simulink model "MPPT"  (R2024b)
settings: Solver=FixedStepAuto  StartTime=0.0  StopTime=1  FixedStep=Ts  RelTol=1e-3
InitFcn:
  | Ts = 1e-6;
  | N = 1000;
  | A = -0.001;
  | B = 0.001
libraries: simulink x9, spsSeriesRLCBranchLib x4, spsCurrentMeasurementLib x1, spsDiodeLib x1, spsMosfetLib x1, spsPVArrayLib x1, spsVoltageMeasurementLib x1, sps_lib x1
settings Model: Creator=Ketan  LastModifiedBy=Ketan

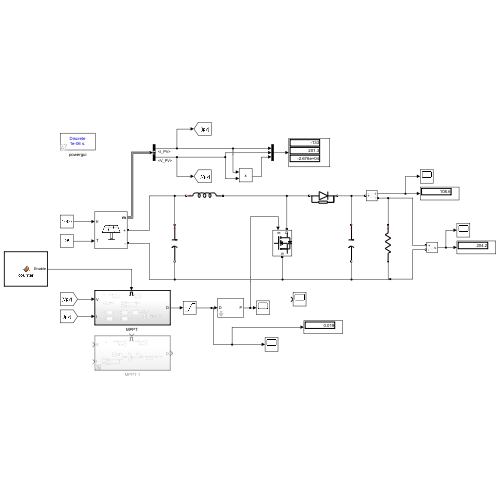
[thumbnail: Simulink's stored preview of the top-level diagram]
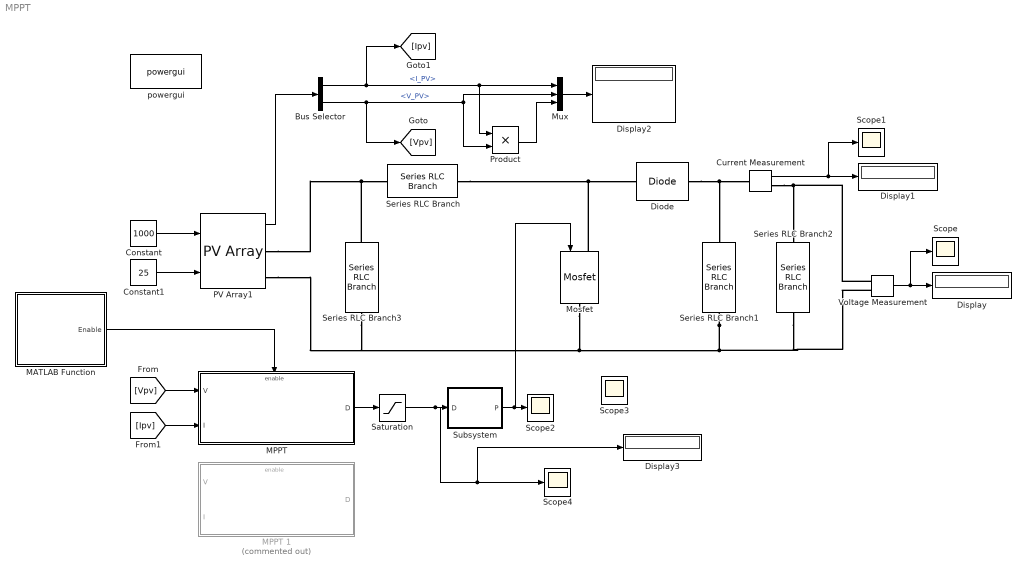
== system MPPT ==
  Bus Selector : BusSelector  OutputSignals=I_PV,V_PV
  Constant : Constant  Value=1000
  Constant1 : Constant  Value=25
  Current Measurement : spsCurrentMeasurementLib/Current Measurement  PhasorSimulation=off  OutputType=Complex  PSBequivalent=0
  Diode : spsDiodeLib/Diode  Ron=0.001  Lon=0  Vf=0.8  IC=0  UseSnubber=0  Rs=500  Cs=250e-9  Measurements=off
  Display{,1..3} (4 alike) : Display
  MATLAB Function : MATLAB Function  TreatAsAtomicUnit=on
  "MPPT " : Subsystem
  MPPT 1 : Subsystem  Commented=on
  Mosfet : spsMosfetLib/Mosfet  Ron=0.1  Lon=0  Rd=0.01  Vfd=0  IC=0  Rs=1e5  Cs=inf  Measurements=off
  Mux : Mux  Inputs=3
  PV Array1 : spsPVArrayLib/PV Array  Npar=40  Nser=10  PlotType=array @ 1000 W/m2 & specified temperatures  S_vec="[ 1000  500  100 ]"  Temp_C_vec="[ 45 25  ]"  ModuleName=User-defined  PlotWhenSelected=off  Pm=213.15  Ncell=60  Voc=36.3  Isc=7.84  Vm=29  Im=7.35  beta_Voc_pc=-0.36099  alpha_Isc_pc=0.102  beta_Voc=-0.13104  alpha_Isc=0.0079968  IL=7.8654  I0=2.9273e-10  nI=0.98119  Rsh=313.0553  Rs=0.39381  RobustModel=off  RobustCellTemperature=313.3991  BAL=on  Tc=1e-6  Tfilter=5e-5
  Product : Product
  Saturation : Saturate  UpperLimit=0.9  LowerLimit=0.005
  Scope{,1..4} (5 alike) : Scope
  Series RLC Branch : spsSeriesRLCBranchLib/Series RLC Branch  LConnTagsString=__new0  RConnTagsString=__new0  BranchType=L  Resistance=1  Inductance=45e-6  SetiL0=off  InitialCurrent=0  Capacitance=1e-6  Setx0=off  InitialVoltage=0  Measurements=None
  Series RLC Branch1 : spsSeriesRLCBranchLib/Series RLC Branch  LConnTagsString=__new0  RConnTagsString=__new0  BranchType=C  Resistance=1  Inductance=1e-3  SetiL0=off  InitialCurrent=0  Capacitance=244e-6  Setx0=off  InitialVoltage=400  Measurements=None
  Series RLC Branch2 : spsSeriesRLCBranchLib/Series RLC Branch  LConnTagsString=__new0  RConnTagsString=__new0  BranchType=R  Resistance=1.88  Inductance=1e-3  SetiL0=off  InitialCurrent=0  Capacitance=1e-6  Setx0=off  InitialVoltage=0  Measurements=None
  Series RLC Branch3 : spsSeriesRLCBranchLib/Series RLC Branch  LConnTagsString=__new0  RConnTagsString=__new0  BranchType=C  Resistance=1  Inductance=1e-3  SetiL0=off  InitialCurrent=0  Capacitance=100e-6  Setx0=off  InitialVoltage=0  Measurements=None
  Subsystem : Subsystem  mask{fs=20000}
      mask prompts: fs "Frequency"
      mask DialogControl DescTextVar Prompt: This Block Genertates a PWM signal based on the Frequency of Carrier Wave and Duty Cycle
  Voltage Measurement : spsVoltageMeasurementLib/Voltage Measurement  PhasorSimulation=off  OutputType=Complex  PSBequivalent=0
  powergui : sps_lib/powergui  Priority=1  SimulationMode=Discrete  SampleTime=Ts  frequency=60  Iterations=50  frequencyindice=0  Pbase=100e6  ErrMax=1e-4  UnitsV=kV  UnitsW=MW  buscounter=0  FunctionMessages=off  echomessages=off  EnableUseOfTLC=off  CurrentSourceSwitches=off  DisableSnubberDevices=off  DisableRonSwitches=off  DisableVfSwitches=off  DisplayEquations=off  AutomaticDiscreteSolvers=off  SolverType=Tustin/Backward Euler (TBE)  Interpol=off  ExternalGateDelay=off  methode=off  Ts=100  x0status=blocks  SPID=on  SwTol=0  HookPort=off  NonlinearTolerance=1e-4  nMaxIteration=100  ContinueOnMaxIteration=off  RestoreLinks=warning  ResistiveCurrentMeasurement=off  Frange=[0:2:500]  Ylog=off  Xlog=on  ShowGrid=off  save=off  variable=ZData  structure=0  ZoomFFT=off  StartTime=0.0  cycles=1  DisplayStyle=1  fundamental=60  FreqAxis=off  MaxFrequency=1000  frequencyindicesteady=1  RmsSteady=1  display=off
  wires:
  Voltage Measurement/1 -> Scope/1, Display/1
  Subsystem/1(P) -> Mosfet/1, Scope2/1
  Constant/1 -> PV Array1/1
  Constant1/1 -> PV Array1/2
  PV Array1/1 -> Bus Selector/1
  Mux/1 -> Display2/1
  Current Measurement/1 -> Scope1/1, Display1/1
  Saturation/1 -> Display3/1, Scope4/1, Subsystem/1(D)
  Bus Selector/1 -> [Ipv], Product/1, Mux/1  "<I_PV>"
  Bus Selector/2 -> [Vpv], Product/2, Mux/2  "<V_PV>"
  "MPPT "/1(D) -> Saturation/1
  MATLAB Function/1(Enable) -> "MPPT "/Enable
  [Vpv] -> "MPPT "/1(V)
  [Ipv] -> "MPPT "/2(I)
  Product/1 -> Mux/3
  connections:
  Series RLC Branch1/RConn1 -- Voltage Measurement/LConn2 -- Series RLC Branch2/RConn1 -- Series RLC Branch3/RConn1 -- PV Array1/RConn2 -- Mosfet/RConn1
  Mosfet/LConn1 -- Series RLC Branch/RConn1 -- Diode/LConn1
  Diode/RConn1 -- Current Measurement/LConn1 -- Series RLC Branch1/LConn1
  PV Array1/RConn1 -- Series RLC Branch3/LConn1 -- Series RLC Branch/LConn1
  Voltage Measurement/LConn1 -- Current Measurement/RConn1 -- Series RLC Branch2/LConn1

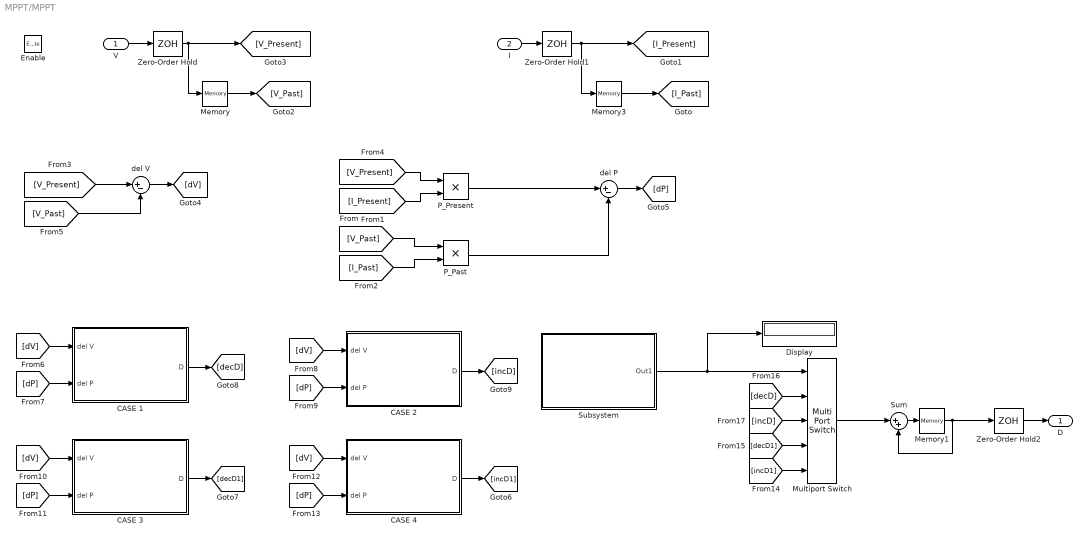
== system MPPT/MPPT  ==
  V : Inport
  I : Inport  Port=2
  Enable : EnablePort
  CASE 1 : Subsystem
  CASE 2 : Subsystem
  CASE 3 : Subsystem
  CASE 4 : Subsystem
  Display : Display
  Memory : Memory
  Memory1 : Memory
  Memory3 : Memory
  Multiport Switch : MultiPortSwitch  Inputs=4  SaturateOnIntegerOverflow=off  InputSameDT=off
  P_Past : Product
  P_Present : Product
  Subsystem : Subsystem
  Sum : Sum  Inputs=|++
  Zero-Order Hold : ZeroOrderHold  SampleTime=Ts
  Zero-Order Hold1 : ZeroOrderHold  SampleTime=Ts
  Zero-Order Hold2 : ZeroOrderHold  SampleTime=Ts
  del P : Sum  Inputs=|+-
  del V : Sum  Inputs=|+-
  D : Outport
  wires:
  P_Past/1 -> del P/2
  P_Present/1 -> del P/1
  [V_Past] -> del V/2
  [V_Present] -> del V/1
  [I_Past] -> P_Past/2
  [I_Present] -> P_Present/2
  [V_Past] -> P_Past/1
  [V_Present] -> P_Present/1
  Zero-Order Hold/1 -> [V_Present], Memory/1
  Memory/1 -> [V_Past]
  Zero-Order Hold1/1 -> [I_Present], Memory3/1
  Memory3/1 -> [I_Past]
  I/1 -> Zero-Order Hold1/1
  V/1 -> Zero-Order Hold/1
  del V/1 -> [dV]
  [dV] -> CASE 1/1(del V)
  del P/1 -> [dP]
  [dP] -> CASE 1/2(del P)
  [dV] -> CASE 2/1(del V)
  [dP] -> CASE 2/2(del P)
  [dP] -> CASE 3/2(del P)
  [dV] -> CASE 3/1(del V)
  [dP] -> CASE 4/2(del P)
  [dV] -> CASE 4/1(del V)
  CASE 4/1(D) -> [incD1]
  [incD1] -> Multiport Switch/5
  CASE 3/1(D) -> [decD1]
  [decD1] -> Multiport Switch/4
  CASE 1/1(D) -> [decD]
  [decD] -> Multiport Switch/2
  CASE 2/1(D) -> [incD]
  [incD] -> Multiport Switch/3
  Subsystem/1(Out1) -> Display/1, Multiport Switch/1
  Multiport Switch/1 -> Sum/1
  Sum/1 -> Memory1/1
  Zero-Order Hold2/1 -> D/1
  Memory1/1 -> Sum/2, Zero-Order Hold2/1

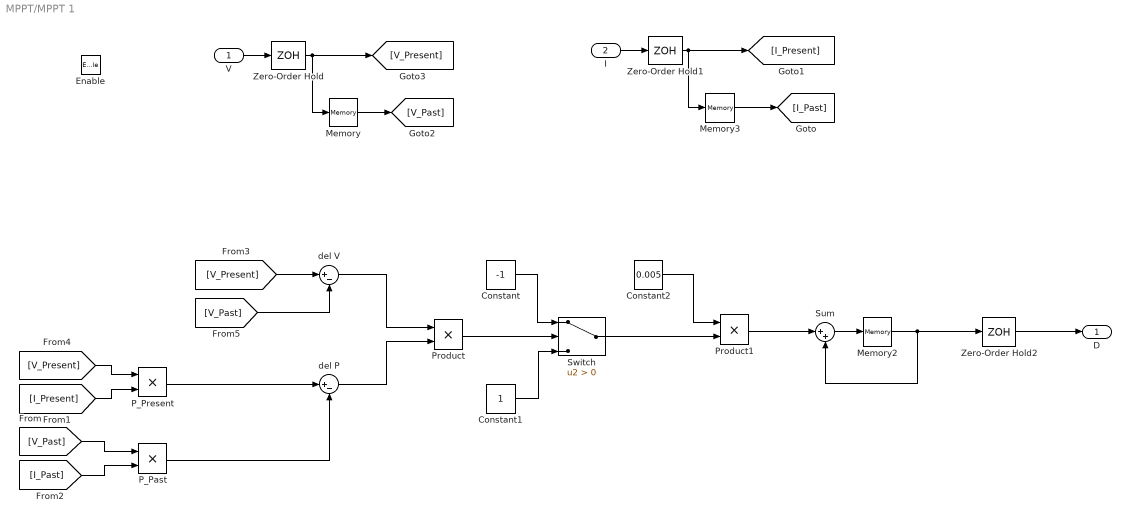
== system MPPT/MPPT 1 ==
  V : Inport
  I : Inport  Port=2
  Enable : EnablePort
  Constant : Constant  Value=-1
  Constant1 : Constant
  Constant2 : Constant  Value=0.005
  Memory : Memory
  Memory2 : Memory
  Memory3 : Memory
  P_Past : Product
  P_Present : Product
  Product : Product
  Product1 : Product
  Sum : Sum  Inputs=|++
  Switch : Switch  Criteria=u2 > Threshold  SaturateOnIntegerOverflow=off  InputSameDT=off
  Zero-Order Hold : ZeroOrderHold  SampleTime=Ts
  Zero-Order Hold1 : ZeroOrderHold  SampleTime=Ts
  Zero-Order Hold2 : ZeroOrderHold  SampleTime=-1
  del P : Sum  Inputs=|+-
  del V : Sum  Inputs=|+-
  D : Outport
  wires:
  V/1 -> Zero-Order Hold/1
  I/1 -> Zero-Order Hold1/1
  Memory3/1 -> [I_Past]
  Zero-Order Hold1/1 -> Memory3/1, [I_Present]
  Memory/1 -> [V_Past]
  Zero-Order Hold/1 -> Memory/1, [V_Present]
  [V_Present] -> P_Present/1
  [V_Past] -> P_Past/1
  [I_Present] -> P_Present/2
  [I_Past] -> P_Past/2
  [V_Present] -> del V/1
  [V_Past] -> del V/2
  P_Present/1 -> del P/1
  P_Past/1 -> del P/2
  del V/1 -> Product/1
  del P/1 -> Product/2
  Product/1 -> Switch/2
  Constant/1 -> Switch/1
  Constant1/1 -> Switch/3
  Switch/1 -> Product1/2
  Constant2/1 -> Product1/1
  Product1/1 -> Sum/1
  Sum/1 -> Memory2/1
  Memory2/1 -> Sum/2, Zero-Order Hold2/1
  Zero-Order Hold2/1 -> D/1

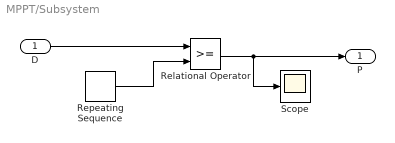
== system MPPT/Subsystem ==
  D : Inport
  Relational Operator : RelationalOperator  OutDataTypeStr=boolean  RndMeth=Simplest  InputSameDT=off
  Repeating Sequence : simulink/Sources/Repeating Sequence  rep_seq_t=[0 1/fs]  rep_seq_y=[0 1]
  Scope : Scope
  P : Outport
  wires:
  D/1 -> Relational Operator/1
  Repeating Sequence/1 -> Relational Operator/2
  Relational Operator/1 -> Scope/1, P/1

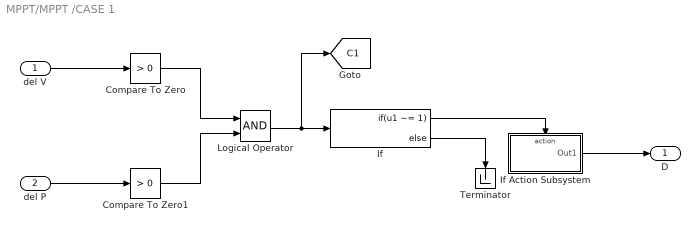
== system MPPT/MPPT /CASE 1 ==
  del V : Inport
  del P : Inport  Port=2
  Compare To Zero : simulink/Logic and Bit Operations/Compare To Zero  relop=>  OutDataTypeStr=boolean
  Compare To Zero1 : simulink/Logic and Bit Operations/Compare To Zero  relop=>  OutDataTypeStr=boolean
  If : If  IfExpression=u1 ~= 1
  If Action Subsystem : Subsystem  TreatAsAtomicUnit=on
  Logical Operator : Logic  AllPortsSameDT=off  OutDataTypeStr=boolean
  Terminator : Terminator
  D : Outport
  tag scope: C1=global
  wires:
  Compare To Zero1/1 -> Logical Operator/2
  del V/1 -> Compare To Zero/1
  If/1 -> If Action Subsystem/Action
  Logical Operator/1 -> [C1], If/1
  If Action Subsystem/1(Out1) -> D/1
  Compare To Zero/1 -> Logical Operator/1
  If/2 -> Terminator/1
  del P/1 -> Compare To Zero1/1

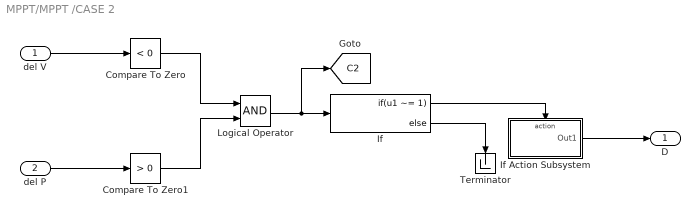
== system MPPT/MPPT /CASE 2 ==
  del V : Inport
  del P : Inport  Port=2
  Compare To Zero : simulink/Logic and Bit Operations/Compare To Zero  relop=<  OutDataTypeStr=boolean
  Compare To Zero1 : simulink/Logic and Bit Operations/Compare To Zero  relop=>  OutDataTypeStr=boolean
  If : If  IfExpression=u1 ~= 1
  If Action Subsystem : Subsystem  TreatAsAtomicUnit=on
  Logical Operator : Logic  AllPortsSameDT=off  OutDataTypeStr=boolean
  Terminator : Terminator
  D : Outport
  tag scope: C2=global
  wires:
  del P/1 -> Compare To Zero1/1
  If/2 -> Terminator/1
  Compare To Zero/1 -> Logical Operator/1
  If Action Subsystem/1(Out1) -> D/1
  Logical Operator/1 -> [C2], If/1
  If/1 -> If Action Subsystem/Action
  del V/1 -> Compare To Zero/1
  Compare To Zero1/1 -> Logical Operator/2

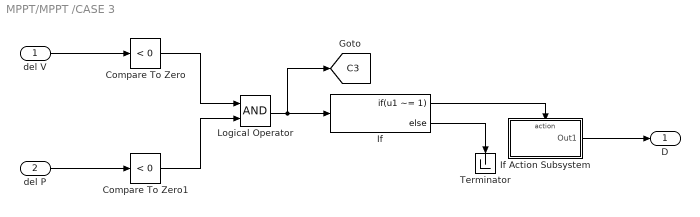
== system MPPT/MPPT /CASE 3 ==
  del V : Inport
  del P : Inport  Port=2
  Compare To Zero : simulink/Logic and Bit Operations/Compare To Zero  relop=<  OutDataTypeStr=boolean
  Compare To Zero1 : simulink/Logic and Bit Operations/Compare To Zero  relop=<  OutDataTypeStr=boolean
  If : If  IfExpression=u1 ~= 1
  If Action Subsystem : Subsystem  TreatAsAtomicUnit=on
  Logical Operator : Logic  AllPortsSameDT=off  OutDataTypeStr=boolean
  Terminator : Terminator
  D : Outport
  tag scope: C3=global
  wires:
  Compare To Zero1/1 -> Logical Operator/2
  del V/1 -> Compare To Zero/1
  If/1 -> If Action Subsystem/Action
  Logical Operator/1 -> [C3], If/1
  If Action Subsystem/1(Out1) -> D/1
  Compare To Zero/1 -> Logical Operator/1
  If/2 -> Terminator/1
  del P/1 -> Compare To Zero1/1

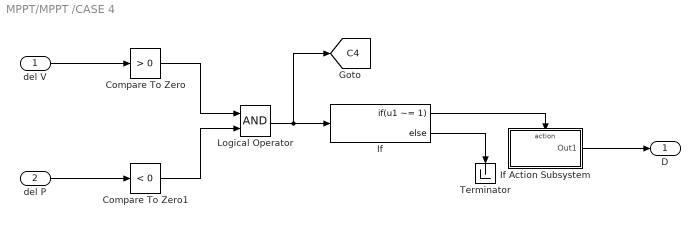
== system MPPT/MPPT /CASE 4 ==
  del V : Inport
  del P : Inport  Port=2
  Compare To Zero : simulink/Logic and Bit Operations/Compare To Zero  relop=>  OutDataTypeStr=boolean
  Compare To Zero1 : simulink/Logic and Bit Operations/Compare To Zero  relop=<  OutDataTypeStr=boolean
  If : If  IfExpression=u1 ~= 1
  If Action Subsystem : Subsystem  TreatAsAtomicUnit=on
  Logical Operator : Logic  AllPortsSameDT=off  OutDataTypeStr=boolean
  Terminator : Terminator
  D : Outport
  tag scope: C4=global
  wires:
  del P/1 -> Compare To Zero1/1
  If/2 -> Terminator/1
  Compare To Zero/1 -> Logical Operator/1
  If Action Subsystem/1(Out1) -> D/1
  Logical Operator/1 -> [C4], If/1
  If/1 -> If Action Subsystem/Action
  del V/1 -> Compare To Zero/1
  Compare To Zero1/1 -> Logical Operator/2

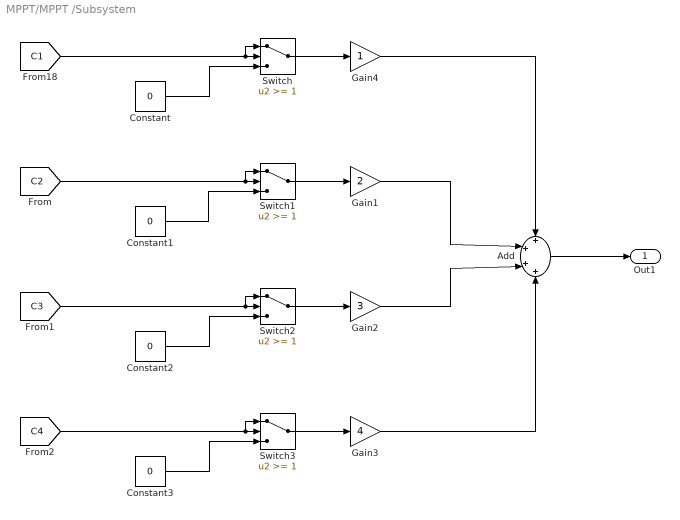
== system MPPT/MPPT /Subsystem ==
  Add : Sum  Inputs=++++
  Constant{,1..3} (4 alike) : Constant  Value=0
  Gain1 : Gain  Gain=2
  Gain2 : Gain  Gain=3
  Gain3 : Gain  Gain=4
  Gain4 : Gain
  Switch{,1..3} (4 alike) : Switch  Threshold=1  SaturateOnIntegerOverflow=off  InputSameDT=off
  Out1 : Outport
  wires:
  [C1] -> Switch/1, Switch/2
  Constant/1 -> Switch/3
  Constant1/1 -> Switch1/3
  [C2] -> Switch1/1, Switch1/2
  Switch1/1 -> Gain1/1
  Switch2/1 -> Gain2/1
  [C3] -> Switch2/2, Switch2/1
  Constant2/1 -> Switch2/3
  Constant3/1 -> Switch3/3
  [C4] -> Switch3/1, Switch3/2
  Switch3/1 -> Gain3/1
  Switch/1 -> Gain4/1
  Gain4/1 -> Add/1
  Gain1/1 -> Add/2
  Gain2/1 -> Add/3
  Gain3/1 -> Add/4
  Add/1 -> Out1/1

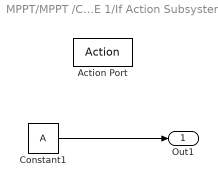
== system MPPT/MPPT /CASE 1/If Action Subsystem ==
  Action Port : ActionPort  ActionPortLabel=if(u1 ~= 1)
  Constant1 : Constant  Value=A
  Out1 : Outport
  wires:
  Constant1/1 -> Out1/1

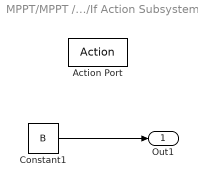
== system MPPT/MPPT /CASE 2/If Action Subsystem ==
  Action Port : ActionPort  ActionPortLabel=if(u1 ~= 1)
  Constant1 : Constant  Value=B
  Out1 : Outport
  wires:
  Constant1/1 -> Out1/1

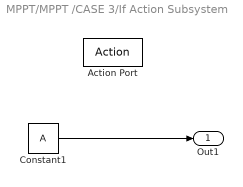
== system MPPT/MPPT /CASE 3/If Action Subsystem ==
  Action Port : ActionPort  ActionPortLabel=if(u1 ~= 1)
  Constant1 : Constant  Value=A
  Out1 : Outport
  wires:
  Constant1/1 -> Out1/1

== system MPPT/MPPT /CASE 4/If Action Subsystem ==
  Action Port : ActionPort  ActionPortLabel=if(u1 ~= 1)
  Constant1 : Constant  Value=B
  Out1 : Outport
  wires:
  Constant1/1 -> Out1/1

== matlab function MPPT/MATLAB Function ==
  data: Enable output
function Enable  = counter
    persistent n
    if isempty(n)
        n = 0;
    end

    n = n + 1;
    if n >= 1000

        Enable = 1;
        n = 0;
    else
       
        Enable = 0;
    end
end
